simulink model "Problem5_27_BlockDiagram"  (R2020b)
settings: Solver=VariableStepAuto  StartTime=0.0  StopTime=10.0  RelTol=1e-3
model workspace: external: MAT-File /Users/jonathanmoran/Development/MAE143B-Linear-Control/5-State-Space-Models-and-Linearization/Problem5_27.mat (data not in the file)
values from neighbouring files (symbols this model uses):
  b_1 = 0.1    [Problem5_27.m]
  b_2 = b_1    (= 0.1)    [Problem5_27.m]
  k_1 = 1    [Problem5_27.m]
  k_2 = 2    [Problem5_27.m]
  m_1 = 1    [Problem5_27.m]
  m_2 = m_1    (= 1)    [Problem5_27.m]
  x_1_init = 0    [Problem5_27.m]    (also in Problem5_48.m = 9)
  x_2_init = 0    [Problem5_27.m]    (also in Problem5_48.m = 1)
settings Model: OrderedModelArguments=off  Creator=jonathanmoran  LastModifiedBy=jonathanmoran
settings DataIOCC: InspectSignalLogs=on

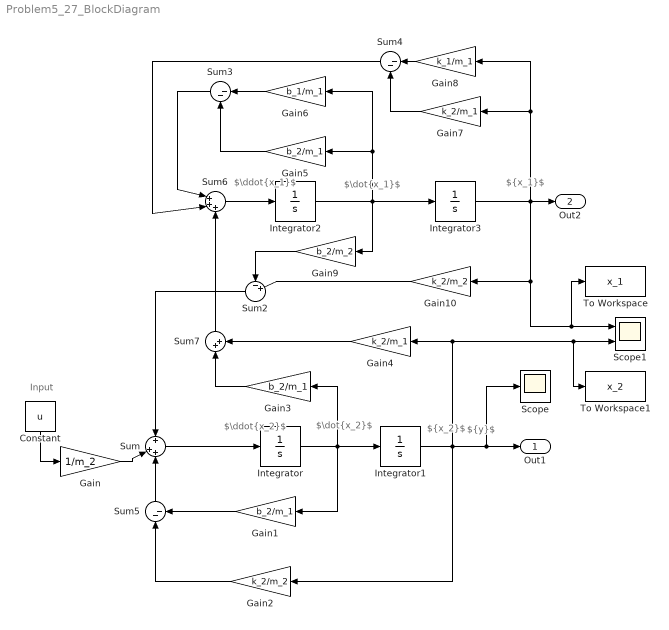
== system Problem5_27_BlockDiagram ==
  note: $\ddot{x_2}$
  note: Input
  note: $\dot{x_2}$
  note: ${x_2}$
  note: $\dot{x_1}$
  note: $\ddot{x_1}$
  note: ${x_1}$
  note: ${y}$
  Constant : Constant  Value=u
  Gain : Gain  Gain=1/m_2
  Gain1 : Gain  Gain=b_2/m_1
  Gain10 : Gain  Gain=k_2/m_2
  Gain2 : Gain  Gain=k_2/m_2
  Gain3 : Gain  Gain=b_2/m_1
  Gain4 : Gain  Gain=k_2/m_1
  Gain5 : Gain  Gain=b_2/m_1
  Gain6 : Gain  Gain=b_1/m_1
  Gain7 : Gain  Gain=k_2/m_1
  Gain8 : Gain  Gain=k_1/m_1
  Gain9 : Gain  Gain=b_2/m_2
  Integrator : Integrator  InitialCondition=x_2_init
  Integrator1 : Integrator  InitialCondition=x_2_init
  Integrator2 : Integrator  InitialCondition=x_1_init
  Integrator3 : Integrator  InitialCondition=x_1_init
  Scope : Scope
  Scope1 : Scope  NumInputPorts=2
  Sum : Sum  Inputs=+|++
  Sum2 : Sum  Inputs=-+||
  Sum3 : Sum  Inputs=|--
  Sum4 : Sum  Inputs=|--
  Sum5 : Sum  Inputs=|--
  Sum6 : Sum  Inputs=|+++
  Sum7 : Sum  Inputs=|++
  To Workspace : ToWorkspace  VariableName=x_1  SampleTime=-1
  To Workspace1 : ToWorkspace  VariableName=x_2  SampleTime=-1
  Out1 : Outport  SignalName=y
  Out2 : Outport  Port=2  SignalName=y
  wires:
  Gain/1 -> Sum/2
  Sum/1 -> Integrator/1
  Integrator/1 -> Gain3/1, Integrator1/1, Gain1/1
  Gain1/1 -> Sum5/2
  Gain2/1 -> Sum5/1
  Sum5/1 -> Sum/3
  Gain3/1 -> Sum7/1
  Gain4/1 -> Sum7/2
  Sum6/1 -> Integrator2/1
  Integrator2/1 -> Gain9/1, Gain6/1, Gain5/1, Integrator3/1
  Gain10/1 -> Sum2/2
  Gain9/1 -> Sum2/1
  Sum2/1 -> Sum/1
  Sum7/1 -> Sum6/3
  Gain5/1 -> Sum3/2
  Gain6/1 -> Sum3/1
  Sum3/1 -> Sum6/1
  Gain7/1 -> Sum4/2
  Gain8/1 -> Sum4/1
  Sum4/1 -> Sum6/2
  Constant/1 -> Gain/1
  Integrator1/1 -> Scope/1, Out1/1, Gain4/1, To Workspace1/1, Scope1/2, Gain2/1
  Integrator3/1 -> Out2/1, Gain7/1, Gain8/1, To Workspace/1, Scope1/1, Gain10/1
